simulink model "Subsystems_merged"  (R2018b)
settings: Solver=FixedStepDiscrete  StartTime=0.0  StopTime=20  FixedStep=1e-07  RelTol=1e-3
undefined symbols (not defined in the file): Acid, Lead
libraries: powerlib x23, electricdrivelib x1, powerlib_meascontrol x1, pePwmGenerator x1
settings Model: SimulationMode=accelerator  Creator=ayaz  LastModifiedBy=defne
settings DataIOCC: ReturnWorkspaceOutputs=on

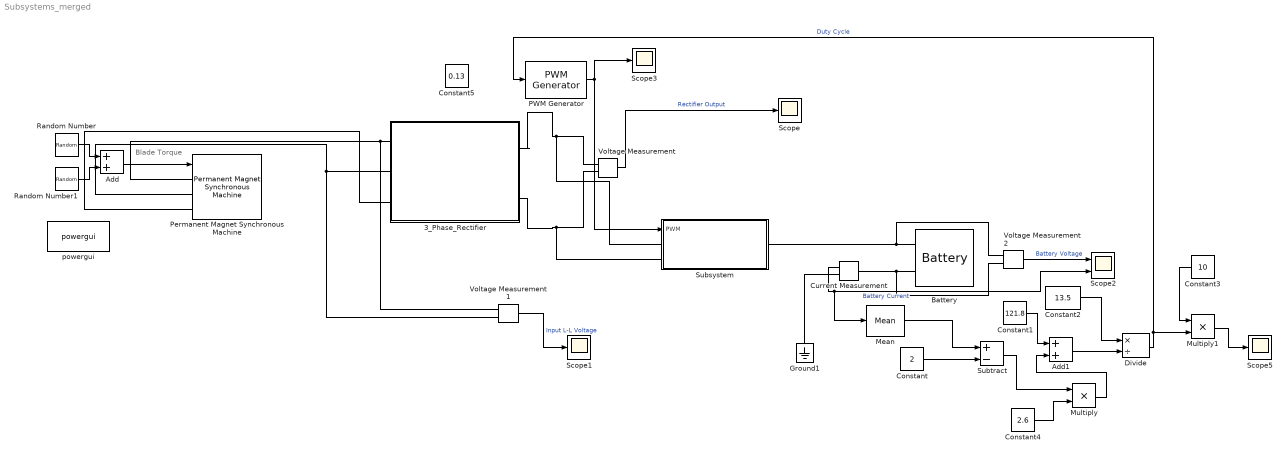
== system Subsystems_merged ==
  note: Blade Torque
  3_Phase_Rectifier : Subsystem
  Add : Sum
  Add1 : Sum
  Battery : electricdrivelib/Extra Sources/Battery  BatType=Lead-Acid  ShowTempParam=off  ThermalPreset=no  ShowAgeParam=off  NomV=24  NomQ=5.4  SOC=50  Batt_Tr=30  PresetModel=on  MaxQ=5.625  MinV=18  FullV=26.1316  Dis_rate=1.08  R=0.044444  Normal_OP=1.6755  expZone="[24.4342        0.018]"  current=[6.5 13 32.5]  Units=Time  Tci=20  NomT=20  T2=-30  MaxQ2=4.8  FullV2=7.1  Normal_OP2=5.655  expZone2="[6.58           1]"  Rca=0.6  ti=2000  Dp=0  Neq0=0  Tsim=1e6  Ta1=25  Qeol=5.4*0.9  Reol=0.013333*1.2  Char_age=[2.3478, 3]  Dis_age=[2.3478, 10]  N1=1500  N2=10500  N3=1000  N4=1400  Ta2=45  N5=950
      settings: SourceProductName=Simscape Electrical
  Constant : Constant  Value=2
  Constant1 : Constant  Value=121.8
  Constant2 : Constant  Value=13.5
  Constant3 : Constant  Value=10
  Constant4 : Constant  Value=2.6
  Constant5 : Constant  Value=0.13
  Current Measurement : powerlib/Measurements/Current Measurement  PhasorSimulation=off  OutputType=Complex  PSBequivalent=0
      settings: SourceProductName=Simscape Electrical
  Divide : Product  Inputs=*/
  Ground1 : powerlib/Elements/Ground  LConnTagsString=a
      settings: SourceProductName=Simscape Electrical
  Mean : powerlib_meascontrol/Measurements/Mean  Freq=10000  Vinit=0  Ts=1e-5
      settings: SourceProductName=Simscape Electrical
  Multiply : Product
  Multiply1 : Product
  PWM Generator : pePwmGenerator/PWM Generator  CarrCount=Up  Tper=0.0001  Ts=1e-5
  Permanent Magnet Synchronous Machine : powerlib/Machines/Permanent Magnet Synchronous Machine  NbPhases=3  FluxDistribution=Sinusoidal  RotorType=Round  MechanicalLoad=Torque Tm  PresetModel=No  ShowDetailedParameters=on  MeasurementBus=off  Resistance=10.58  Inductance=8.5e-3  dqInductances=[8.5e-3,8.5e-3]  La=0.0167  MachineConstant=Voltage Constant (V_peak L-L / krpm)  Flux=0.60646  VoltageCst=110  TorqueCst=0.90969  Flat=120  Mechanical=[0.00027 0.005024 1 0]  PolePairs=4  InitialConditions=[300,0, 0,0]  InitialConditions5ph=[0 0 0 0 0 0]  TsPowergui=0  TsBlock=-1  RefAngle=90 degrees behind phase A axis (modified Park)
  Random Number : RandomNumber  Mean=-1.6  Variance=0.05  SampleTime=1
  Random Number1 : RandomNumber  Variance=0.1  SampleTime=1e-3
  Scope{,1,3,5} (4 alike) : Scope
  Scope2 : Scope  NumInputPorts=2
  Subsystem : Subsystem
  Subtract : Sum  Inputs=+-
  Voltage Measurement : powerlib/Measurements/Voltage Measurement  PhasorSimulation=off  OutputType=Complex  PSBequivalent=0
      settings: SourceProductName=Simscape Electrical
  Voltage Measurement1 : powerlib/Measurements/Voltage Measurement  PhasorSimulation=off  OutputType=Complex  PSBequivalent=0
      settings: SourceProductName=Simscape Electrical
  Voltage Measurement2 : powerlib/Measurements/Voltage Measurement  PhasorSimulation=off  OutputType=Complex  PSBequivalent=0
      settings: SourceProductName=Simscape Electrical
  powergui : powerlib/powergui  Priority=1  SimulationMode=Discrete  SampleTime=1e-5  frequency=60  Iterations=50  frequencyindice=0  Pbase=100e6  ErrMax=1e-4  UnitsV=kV  UnitsW=MW  buscounter=0  FunctionMessages=off  echomessages=off  EnableUseOfTLC=off  CurrentSourceSwitches=off  DisableSnubberDevices=off  DisableRonSwitches=off  DisableVfSwitches=off  DisplayEquations=off  SolverType=Tustin/Backward Euler (TBE)  Interpol=off  ExternalGateDelay=off  methode=off  Ts=100  x0status=blocks  SPID=on  SwTol=0  HookPort=off  RestoreLinks=warning  ResistiveCurrentMeasurement=off  Frange=[0:2:500]  Ylog=off  Xlog=on  ShowGrid=off  save=off  variable=ZData  structure=0  ZoomFFT=off  StartTime=0.0  cycles=1  DisplayStyle=1  fundamental=60  FreqAxis=off  MaxFrequency=1000  frequencyindicesteady=1  RmsSteady=1  display=off
      settings: SourceProductName=Simscape Electrical
  wires:
  Random Number/1 -> Add/1
  Random Number1/1 -> Add/2
  Add/1 -> Permanent Magnet Synchronous Machine/1
  Voltage Measurement/1 -> Scope/1  "Rectifier Output"
  Voltage Measurement1/1 -> Scope1/1  "Input L-L Voltage"
  PWM Generator/1 -> Scope3/1, Subsystem/1(PWM)
  Voltage Measurement2/1 -> Scope2/1  "Battery Voltage"
  Current Measurement/1 -> Mean/1, Scope2/2  "Battery Current"
  Constant/1 -> Subtract/2
  Constant1/1 -> Add1/1
  Add1/1 -> Divide/2
  Constant2/1 -> Divide/1
  Subtract/1 -> Multiply/1
  Constant4/1 -> Multiply/2
  Multiply/1 -> Add1/2
  Divide/1 -> Multiply1/2, PWM Generator/1  "Duty Cycle"
  Constant3/1 -> Multiply1/1
  Multiply1/1 -> Scope5/1
  Mean/1 -> Subtract/1
  connections:
  Permanent Magnet Synchronous Machine/LConn1 -- Voltage Measurement1/LConn1 -- 3_Phase_Rectifier/LConn1
  Permanent Magnet Synchronous Machine/LConn3 -- 3_Phase_Rectifier/LConn3
  3_Phase_Rectifier/RConn1 -- Subsystem/LConn1 -- Voltage Measurement/LConn1
  Voltage Measurement/LConn2 -- Subsystem/LConn2 -- 3_Phase_Rectifier/RConn2
  Permanent Magnet Synchronous Machine/LConn2 -- Voltage Measurement1/LConn2 -- 3_Phase_Rectifier/LConn2
  Voltage Measurement2/LConn1 -- Subsystem/RConn1 -- Battery/LConn1
  Voltage Measurement2/LConn2 -- Battery/LConn2 -- Current Measurement/LConn1
  Ground1/LConn1 -- Current Measurement/RConn1

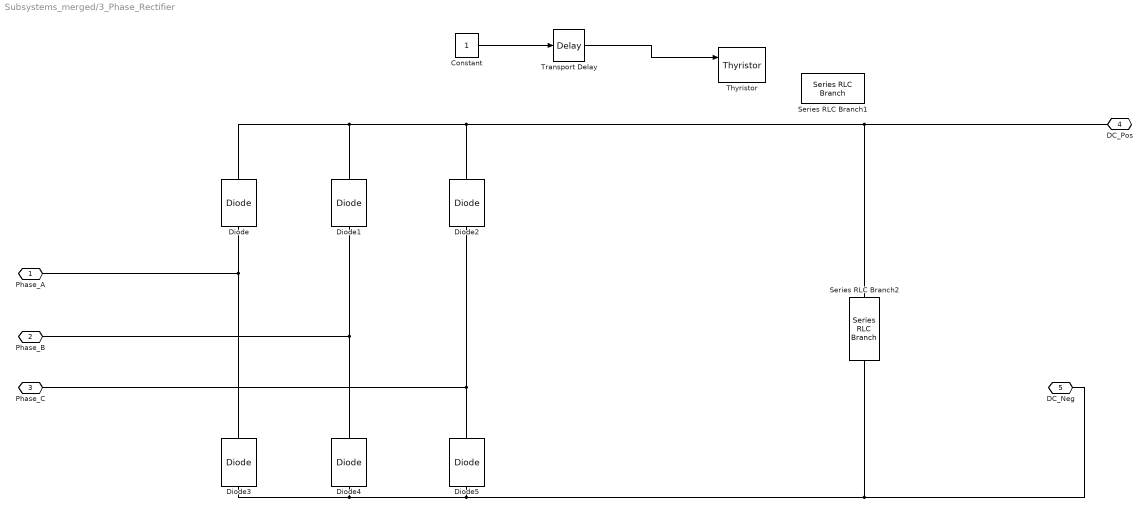
== system Subsystems_merged/3_Phase_Rectifier ==
  Constant : Constant
  Diode{,1..5} (6 alike) : powerlib/Power Electronics/Diode  Ron=0.001  Lon=0  Vf=0.8  IC=0  UseSnubber=0  Rs=500  Cs=250e-9  Measurements=off
      settings: SourceProductName=Simscape Electrical
  Series RLC Branch1 : powerlib/Elements/Series RLC Branch  LConnTagsString=__new0  RConnTagsString=__new0  BranchType=R  Resistance=1000  Inductance=1e-3  SetiL0=off  InitialCurrent=0  Capacitance=1e-6  Setx0=off  InitialVoltage=0  Measurements=None
      settings: SourceProductName=Simscape Electrical
  Series RLC Branch2 : powerlib/Elements/Series RLC Branch  LConnTagsString=__new0  RConnTagsString=__new0  BranchType=C  Resistance=72  Inductance=1e-3  SetiL0=off  InitialCurrent=0  Capacitance=4e-3  Setx0=off  InitialVoltage=0  Measurements=None
      settings: SourceProductName=Simscape Electrical
  Thyristor : powerlib/Power Electronics/Thyristor  Ron=0.001  Lon=0  Vf=0.8  IC=0  Rs=500  Cs=250e-9  Measurements=off
      settings: SourceProductName=Simscape Electrical
  Transport Delay : TransportDelay  DelayTime=0.2
  Phase_A : PMIOPort  Side=Left
  Phase_B : PMIOPort  Port=2  Side=Left
  Phase_C : PMIOPort  Port=3  Side=Left
  DC_Pos : PMIOPort  Port=4  Side=Right
  DC_Neg : PMIOPort  Port=5  Side=Right
  wires:
  Transport Delay/1 -> Thyristor/1
  Constant/1 -> Transport Delay/1
  connections:
  Diode2/LConn1 -- Phase_C/RConn1 -- Diode5/RConn1
  Series RLC Branch2/LConn1 -- Diode2/RConn1 -- Diode1/RConn1 -- Diode/RConn1 -- DC_Pos/RConn1
  Series RLC Branch2/RConn1 -- Diode3/LConn1 -- Diode4/LConn1 -- Diode5/LConn1 -- DC_Neg/RConn1
  Diode/LConn1 -- Phase_A/RConn1 -- Diode3/RConn1
  Diode4/RConn1 -- Phase_B/RConn1 -- Diode1/LConn1

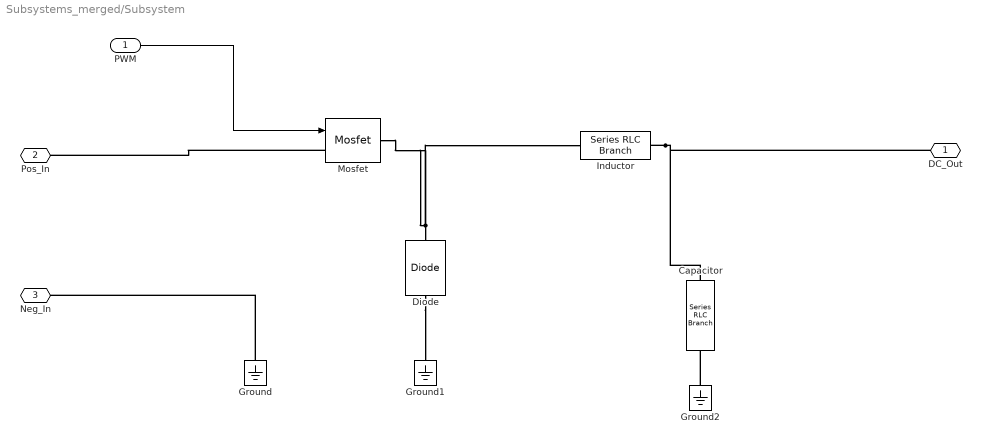
== system Subsystems_merged/Subsystem ==
  PWM : Inport
  Capacitor : powerlib/Elements/Series RLC Branch  LConnTagsString=__new0  RConnTagsString=__new0  BranchType=C  Resistance=1  Inductance=1e-3  SetiL0=off  InitialCurrent=0  Capacitance=4.7e-6  Setx0=off  InitialVoltage=0  Measurements=None
      settings: SourceProductName=Simscape Electrical
  Diode : powerlib/Power Electronics/Diode  Ron=0.001  Lon=0  Vf=0.8  IC=0  UseSnubber=off  Rs=500  Cs=250e-9  Measurements=off
      settings: SourceProductName=Simscape Electrical
  Ground : powerlib/Elements/Ground  LConnTagsString=a
      settings: SourceProductName=Simscape Electrical
  Ground1 : powerlib/Elements/Ground  LConnTagsString=a
      settings: SourceProductName=Simscape Electrical
  Ground2 : powerlib/Elements/Ground  LConnTagsString=a
      settings: SourceProductName=Simscape Electrical
  Inductor : powerlib/Elements/Series RLC Branch  LConnTagsString=__new0  RConnTagsString=__new0  BranchType=L  Resistance=1  Inductance=5e-3  SetiL0=off  InitialCurrent=0  Capacitance=1e-6  Setx0=off  InitialVoltage=0  Measurements=None
      settings: SourceProductName=Simscape Electrical
  Mosfet : powerlib/Power Electronics/Mosfet  Ron=0.1  Lon=0  Rd=0.01  Vfd=0  IC=0  Rs=1e5  Cs=inf  Measurements=off
      settings: SourceProductName=Simscape Electrical
  DC_Out : PMIOPort  Side=Right
  Pos_In : PMIOPort  Port=2  Side=Left
  Neg_In : PMIOPort  Port=3  Side=Left
  wires:
  PWM/1 -> Mosfet/1
  connections:
  Ground2/LConn1 -- Capacitor/RConn1
  Diode/RConn1 -- Mosfet/RConn1 -- Inductor/LConn1
  Inductor/RConn1 -- Capacitor/LConn1 -- DC_Out/RConn1
  Diode/LConn1 -- Ground1/LConn1
  Mosfet/LConn1 -- Pos_In/RConn1
  Ground/LConn1 -- Neg_In/RConn1
